simulink model "stm32f0_adc_demo"  (Simulink 7.3)
settings: Solver=ode3  SolverMode=SingleTasking  StartTime=0.0  StopTime=10.0  RelTol=1e-3
PreLoadFcn:
  | waijung.modelPreload; % Required for working with Waijung Blockset. Do not remove.
undefined symbols (not defined in the file): current, LQFP48, STM32F072CB, voltage
libraries: simulink x2, stm32f0_adc_lib x2, stm32f0_io_lib x1, stm32f0_device_config_lib x1
CloseFcn:
  | waijung.modelClose; % Required for working with Waijung Blockset. Do not remove.
settings Model: Creator=Krisada  LastModifiedBy=Krisada
settings OptimizationCC: OptimizeModelRefInitCode=on  LifeSpan=1
settings HardwareCC: ProdEndianess=LittleEndian  ProdHWDeviceType=ARM Compatible->Cortex - M0  TargetEndianess=LittleEndian  TargetHWDeviceType=ARM Compatible->Cortex - M0
settings RTWCC: SystemTargetFile=stm32f0.tlc  GenerateMakefile=off  TemplateMakefile=ert_default_tmf  Description=STM32F0 Target  ProcessScript=stm32f0_make_rtw_hook
settings CodeAppCC: IgnoreCustomStorageClasses=off
settings STFCustomTargetCC: ModelReferenceCompliant=off  CombineOutputUpdateFcns=on  ERTCustomFileBanners=on  SupportContinuousTime=off  SupportNonInlinedSFcns=off  SystemTargetFile=stm32f0.tlc
settings ERTTargetCC: MultiwordLength=2048  ModelReferenceCompliant=off  ParMdlRefBuildCompliant=off  CompOptLevelCompliant=off  ERTFirstTimeCompliant=off  ModelStepFunctionPrototypeControlCompliant=off  CPPClassGenCompliant=off  InlinedParameterPlacement=NonHierarchical  ERTSrcFileBannerTemplate=stm32f0_code_template.cgt  ERTHdrFileBannerTemplate=stm32f0_code_template.cgt  ERTDataSrcFileTemplate=stm32f0_code_template.cgt  ERTDataHdrFileTemplate=stm32f0_code_template.cgt  ERTCustomFileTemplate=stm32f0_file_process.tlc

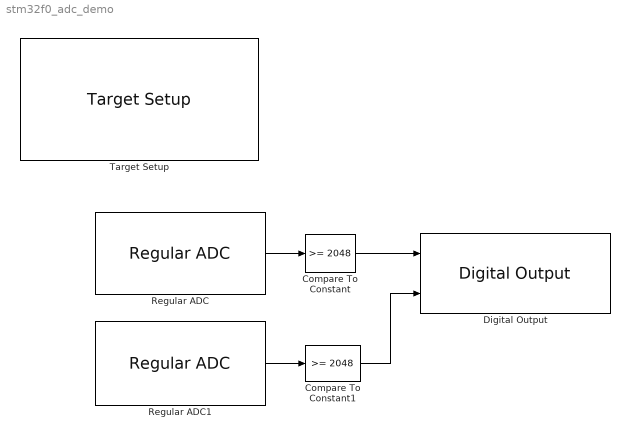
== system stm32f0_adc_demo ==
  Compare To Constant : simulink/Logic and Bit Operations/Compare To Constant  SystemSampleTime=-1  relop=>=  const=2048  LogicOutDataTypeMode=uint8  ZeroCross=off
  Compare To Constant1 : simulink/Logic and Bit Operations/Compare To Constant  SystemSampleTime=-1  relop=>=  const=2048  LogicOutDataTypeMode=uint8  ZeroCross=off
  Digital Output : stm32f0_io_lib/Digital Output  use_bitband=off  port=B  speed=2  porttype=Push Pull  porttypestr=PP  use_pin0=off  use_pin1=off  use_pin2=off  use_pin3=off  use_pin4=off  use_pin5=off  use_pin6=off  use_pin7=off  use_pin8=off  use_pin9=off  use_pin10=off  use_pin11=off  use_pin12=on  use_pin13=on  use_pin14=off  use_pin15=off  pinstr=GPIO_Pin_12 | GPIO_Pin_13  usedpinarray="[0  0  0  0  0  0  0  0  0  0  0  0  1  1  0  0]"  bitbandingstr=|  sampletime=-1  sampletimestr=0.1  blockid=DigitalOutput  enablecustomportlabel=off  cinputportlabel=In1, In2  coutputportlabel=0
      | #define DigitalOutput_B12 Peripheral_BB(GPIOB->ODR, 12)  /* Output pin */
      | #define DigitalOutput_B13 Peripheral_BB(GPIOB->ODR, 13)  /* Output pin */
  Regular ADC : stm32f0_adc_lib/Regular ADC  conf=adc  module=1  samplingtime=239.5 Cycles  outputdatatype=Uint16  adc_ch0=off  adc_ch1=off  adc_ch2=off  adc_ch3=off  adc_ch4=off  adc_ch5=off  adc_ch6=on  adc_ch7=off  adc_ch8=off  adc_ch9=off  adc_ch10=off  adc_ch11=off  adc_ch12=off  adc_ch13=off  adc_ch14=off  adc_ch15=off  adc_ch16=off  adc_ch17=off  adc_ch18=off  sampletime=inf  enablecustomportlabel=off  coutputportlabel=voltage,current  portpinstr=0  blockid=RegularADC  inputporttype=[]  inputportwidth=[]  inputportlabel={}  outputporttype=[5]  outputportwidth=[]  outputportlabel={'ADC_IN6'}  compat=0  optionstring="[\"1\",\"ADC_SampleTime_239_5Cycles\",\"dummy\",\"dummy\",\"dummy\",\"0\",\"A\",\"0\",\"0\",\"A\",\"1\",\"0\",\"A\",\"2\",\"0\",\"A\",\"3\",\"0\",\"A\",\"4\",\"0\",\"A\",\"5\",\"1\",\"A\",\"6\",\"0\",\"A\",\"7\",\"0\",\"B\",\"0\",\"0\",\"B\",\"1\",\"0\",\"C\",\"0\",\"0\",\"C\",\"1\",\"0\",\"C\",\"2\",\"0\",\"C\",\"3\",\"0\",\"C\",\"4\",\"0\",\"C\",\"5\",\"0\",\"A\",\"0\",\"0\",\"A\",\"0\",\"0\",\"A\",\"0\",\"1\",\"1\",\"1\",\"1\",\"0\",\"0\",\"0\",\"uint16_t\"]"
  Regular ADC1 : stm32f0_adc_lib/Regular ADC  conf=adc  module=1  samplingtime=55.5 Cycles  outputdatatype=Uint16  adc_ch0=off  adc_ch1=off  adc_ch2=off  adc_ch3=off  adc_ch4=off  adc_ch5=off  adc_ch6=off  adc_ch7=on  adc_ch8=off  adc_ch9=off  adc_ch10=off  adc_ch11=off  adc_ch12=off  adc_ch13=off  adc_ch14=off  adc_ch15=off  adc_ch16=off  adc_ch17=off  adc_ch18=off  sampletime=inf  enablecustomportlabel=off  coutputportlabel=voltage,current  portpinstr=0  blockid=RegularADC1  inputporttype=[]  inputportwidth=[]  inputportlabel={}  outputporttype=[5]  outputportwidth=[]  outputportlabel={'ADC_IN7'}  compat=0  optionstring="[\"1\",\"ADC_SampleTime_55_5Cycles\",\"dummy\",\"dummy\",\"dummy\",\"0\",\"A\",\"0\",\"0\",\"A\",\"1\",\"0\",\"A\",\"2\",\"0\",\"A\",\"3\",\"0\",\"A\",\"4\",\"0\",\"A\",\"5\",\"0\",\"A\",\"6\",\"1\",\"A\",\"7\",\"0\",\"B\",\"0\",\"0\",\"B\",\"1\",\"0\",\"C\",\"0\",\"0\",\"C\",\"1\",\"0\",\"C\",\"2\",\"0\",\"C\",\"3\",\"0\",\"C\",\"4\",\"0\",\"C\",\"5\",\"0\",\"A\",\"0\",\"0\",\"A\",\"0\",\"0\",\"A\",\"0\",\"1\",\"1\",\"1\",\"1\",\"0\",\"0\",\"0\",\"uint16_t\"]"
  Target Setup : stm32f0_device_config_lib/Target Setup  Priority=100  compiler=GNU ARM  previous_compiler=GNU ARM  mcu=STM32F072CB (LQFP48)  mcustr=STM32F072CB  stdlib=STM32F072  clockconfig=FiO MOTE-ST Default (HSEOSC-8MHz/HCLK-48MHz)  system_stm32f0xx_c_path=F:\trunk\targets\stm32f0_target\stm32f0\utils\STM32F0xx_AN4055\stm32f0_default\hse8mhz_pll_hclk48mhz  showmemoryconfiguration=off  stacksize=0x200  heapsize=0x200  enableautocompiledownload=on  fullchiperase=off  programmerinterface=aMG USB Connect  editctrlstr=on  compilercontrolstr=$(patsubst %, -I%, .) -mcpu=cortex-m0 -mthumb -mabi=aapcs -Wall -O3 -mfloat-abi=soft -ffunction-sections -fdata-sections -fno-strict-aliasing -fno-builtin --short-enums  assemblercontrolstr=$(patsubst %, -I%, .) -mcpu=cortex-m0 -mtune=cortex-m0 -mthumb -Wall -O3 -Wa,-amhls=$(<:.s=.lst) -D__STACK_SIZE=$(STACK_SIZE) -D__HEAP_SIZE=$(HEAP_SIZE)  linkercontrolstr=-T$(LD_SCRIPT) -Wl,-Map=$(MAP),--cref,--no-warn-mismatch -mcpu=cortex-m0 -mthumb -O3 -Wl,--gc-sections --specs=nano.specs -lc -lnosys  runafterdownload=on  execprofile=None  profileruart=3  profilerbaud=500000  profilertxpin=Not used  profilerinitstr=0.1,48000000,4800000,500000,0  manualsetsampletime=off  sampletime=0.1  blockid=TargetSetup  systickreloadvalue=4800000  hseval=8000000  lastprofileruart=3  hclk=48000000  flashorigin=0x8000000  flashlength=128k  ramorigin=0x20000000  ramlength=16k  useextram=off
  wires:
  Regular ADC/1 -> Compare To Constant/1
  Compare To Constant/1 -> Digital Output/1
  Compare To Constant1/1 -> Digital Output/2
  Regular ADC1/1 -> Compare To Constant1/1
